simulink model "Task_3_sim"  (R2023b)
settings: Solver=VariableStepAuto  StartTime=0.0  StopTime=50  RelTol=1e-8
settings Model: Creator=nikita  LastModifiedBy=nikita

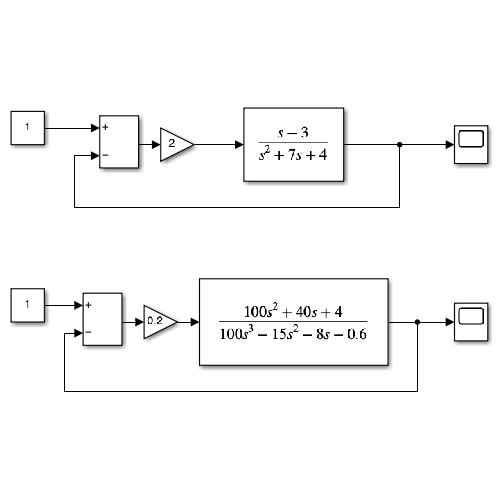
[thumbnail: Simulink's stored preview of the top-level diagram]
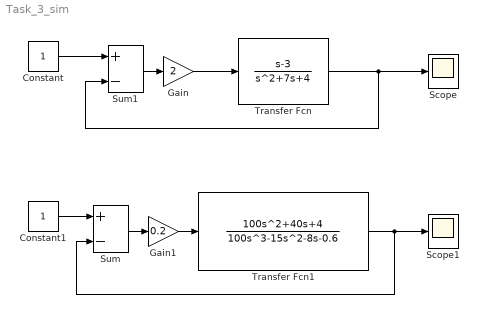
== system Task_3_sim ==
  Constant : Constant
  Constant1 : Constant
  Gain : Gain  Gain=2
  Gain1 : Gain  Gain=0.2
  Scope : Scope
  Scope1 : Scope
  Sum : Sum  Inputs=+-
  Sum1 : Sum  Inputs=+-
  Transfer Fcn : TransferFcn  Numerator=[0 1 -3]  Denominator=[1 7 4]
  Transfer Fcn1 : TransferFcn  Numerator=[100 40 4]  Denominator=[100 -15 -8 -0.6]
  wires:
  Transfer Fcn/1 -> Sum1/2, Scope/1
  Transfer Fcn1/1 -> Sum/2, Scope1/1
  Gain/1 -> Transfer Fcn/1
  Gain1/1 -> Transfer Fcn1/1
  Sum/1 -> Gain1/1
  Constant1/1 -> Sum/1
  Sum1/1 -> Gain/1
  Constant/1 -> Sum1/1
